simulink model "MPPT_Android"  (R2020a)
settings: Solver=FixedStepAuto  StartTime=0.0  StopTime=0.5  RelTol=1e-3
undefined symbols (not defined in the file): Ion, Lithium
libraries: powerlib x40, androiduilib x6, simulink x2, re_lib x2, powerlib_meascontrol x2, electricdrivelib x1, androidadvancedlib x1
settings Model: Creator=kushalgoswami  LastModifiedBy=kushalgoswami
settings OptimizationCC: EnhancedBackFolding=on  PassReuseOutputArgsAs=Individual arguments  ZeroExternalMemoryAtStartup=off  ZeroInternalMemoryAtStartup=off  MaxStackSize=64  OptimizeBlockOrder=speed  DifferentSizesBufferReuse=on  OptimizationCustomize=off  EfficientTunableParamExpr=on
settings DebuggingCC: ParameterTunabilityLossMsg=error
settings HardwareCC: ProdBitPerPointer=32  ProdBitPerSizeT=32  ProdBitPerPtrDiffT=32  ProdLargestAtomicInteger=Long  ProdLargestAtomicFloat=Double  ProdWordSize=32  ProdHWDeviceType=ARM Compatible->ARM Cortex  UseEmbeddedCoderFeatures=off  UseSimulinkCoderFeatures=off
settings SFSimCC: MATLABDynamicMemAlloc=off
settings RTWCC: SystemTargetFile=ert.tlc  HardwareBoard=Android Device  TemplateMakefile=ert_default_tmf  RTWVerbose=off  Toolchain=Android SDK/NDK Tools
settings CodeAppCC: ForceParamTrailComments=on  IgnoreCustomStorageClasses=off  OperatorAnnotations=on  SimulinkDataObjDesc=on  SFDataObjDesc=on  InsertBlockDesc=on
settings ERTTargetCC: SupportNonInlinedSFcns=on

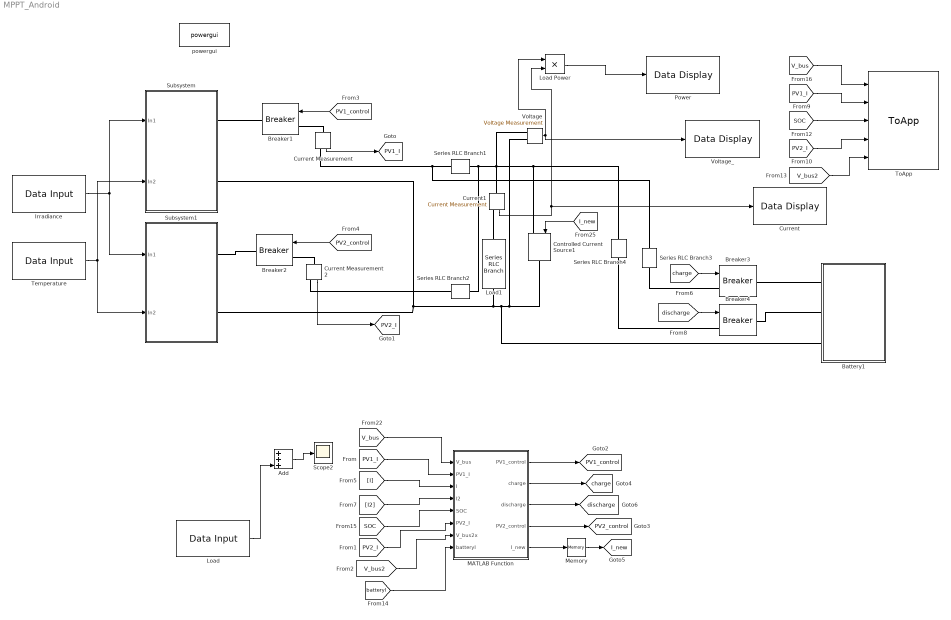
== system MPPT_Android ==
  Add : Sum  Inputs=+++
  Battery1 : Subsystem
  Breaker{1..4} (4 alike) : powerlib/Elements/Breaker  InitialState=0  SwitchingTimes="[1/60  5/60]"  External=on  BreakerResistance=0.01  SnubberResistance=1e6  SnubberCapacitance=inf  Measurements=None  MoreParameters=on  NoBreakLoop=off
  Controlled Current Source1 : powerlib/Electrical Sources/Controlled Current Source  Initialize=off  Source_Type=AC  Amplitude=0  Phase=0  Frequency=0  Measurements=None
  Current : androiduilib/Data Display  DataDisplayId=MPPT_Android/Current  Format=Float  Precision=6  SimulateUsing=Code generation  blockPlatform=Android
      settings: SourceProductBaseCode=ANDROID
  Current Measurement : powerlib/Measurements/Current Measurement  PhasorSimulation=off  OutputType=Complex  PSBequivalent=0
  Current Measurement2 : powerlib/Measurements/Current Measurement  PhasorSimulation=off  OutputType=Complex  PSBequivalent=0
  Current1 : powerlib/Measurements/Current Measurement  PhasorSimulation=off  OutputType=Complex  PSBequivalent=0
  Irradiance : androiduilib/Data Input  isCharVector=off  Value=1000  CharVector=Hello World  OutputDataType=double  maxCharVectorSize=100  DataInputId=MPPT_Android/Irradiance  SampleTime=0.1
      settings: SourceProductBaseCode=ANDROID
  Load : androiduilib/Data Input  isCharVector=off  Value=350  CharVector=Hello World  OutputDataType=double  maxCharVectorSize=100  DataInputId=MPPT_Android/Load  SampleTime=0.1
      settings: SourceProductBaseCode=ANDROID
  Load Power : Product
  Load1 : powerlib/Elements/Series RLC Branch  LConnTagsString=__new0  RConnTagsString=__new0  BranchType=R  Resistance=2  Inductance=1e-3  SetiL0=off  InitialCurrent=0  Capacitance=3300e-6  Setx0=off  InitialVoltage=0  Measurements=None
  MATLAB Function : MATLAB Function  TreatAsAtomicUnit=on
  Memory : Memory
  Power : androiduilib/Data Display  DataDisplayId=MPPT_Android/Power  Format=Float  Precision=6  SimulateUsing=Code generation  blockPlatform=Android
      settings: SourceProductBaseCode=ANDROID
  Scope2 : Scope
  Series RLC Branch{1..4} (4 alike) : powerlib/Elements/Series RLC Branch  LConnTagsString=__new0  RConnTagsString=__new0  BranchType=R  Resistance=0.5  Inductance=1e-3  SetiL0=off  InitialCurrent=0  Capacitance=3300e-6  Setx0=off  InitialVoltage=0  Measurements=None
  Subsystem : Subsystem
      settings: PortSchema="{\"entries\":[{\"content\":{\"sides\":[{\"content\":{\"connectorIds\":[\"LConn1\",\"LConn2\"]},\"type\":\"ConnectorPlacement.EquallySpacedRectSide\",\"uuid\":\"fe52fdc6-6768-4979-b6cd-1f1e64aed3c2\"},{\"content\":{\"connectorIds\":[\"In1\",\"In2\"],\"side\":\"RIGHT\"},\"type\":\"ConnectorPlacement.EquallySpacedRectSide\",\"uuid\":\"5c57de2a-0e2a-4d93-8a44-5c93cac66104\"},{\"content\":{\"connectorIds\":[],\"side\":\"TOP\"},\"type\":\"ConnectorPlacement.EquallySpacedRectSide\",\"uuid\":\"1ec0e451-aef4-49c0-8277-43179a2299e6\"}]},\"type\":\"ConnectorPlacement.EquallySpacedConnector\",\"uuid\":\"46266059-5c92-4136-9283-09609ad0783e\"}],\"packageUris\":[\"http://schema.mathworks.com/mf0/Connector/19700101\"],\"version\":\"1.0\"}"
  Subsystem1 : Subsystem
      settings: PortSchema="{\"entries\":[{\"content\":{\"sides\":[{\"content\":{\"connectorIds\":[\"LConn1\",\"LConn2\"]},\"type\":\"ConnectorPlacement.EquallySpacedRectSide\",\"uuid\":\"fe52fdc6-6768-4979-b6cd-1f1e64aed3c2\"},{\"content\":{\"connectorIds\":[\"In1\",\"In2\"],\"side\":\"RIGHT\"},\"type\":\"ConnectorPlacement.EquallySpacedRectSide\",\"uuid\":\"5c57de2a-0e2a-4d93-8a44-5c93cac66104\"},{\"content\":{\"connectorIds\":[],\"side\":\"TOP\"},\"type\":\"ConnectorPlacement.EquallySpacedRectSide\",\"uuid\":\"1ec0e451-aef4-49c0-8277-43179a2299e6\"}]},\"type\":\"ConnectorPlacement.EquallySpacedConnector\",\"uuid\":\"46266059-5c92-4136-9283-09609ad0783e\"}],\"packageUris\":[\"http://schema.mathworks.com/mf0/Connector/19700101\"],\"version\":\"1.0\"}"
  Temperature : androiduilib/Data Input  isCharVector=off  Value=25  CharVector=Hello World  OutputDataType=double  maxCharVectorSize=100  DataInputId=MPPT_Android/Temperature  SampleTime=0.1
      settings: SourceProductBaseCode=ANDROID
  ToApp : androidadvancedlib/ToApp  FunctionName=ToAppMethod  NumInputs=5
      settings: SourceProductBaseCode=ANDROID
  Voltage : powerlib/Measurements/Voltage Measurement  PhasorSimulation=off  OutputType=Complex  PSBequivalent=0
  Voltage_ : androiduilib/Data Display  DataDisplayId=MPPT_Android/Voltage_  Format=Float  Precision=6  SimulateUsing=Code generation  blockPlatform=Android
      settings: SourceProductBaseCode=ANDROID
  powergui : powerlib/powergui  Priority=1  SimulationMode=Discrete  SampleTime=1e-6  frequency=60  Iterations=50  frequencyindice=0  Pbase=100e6  ErrMax=1e-4  UnitsV=kV  UnitsW=MW  buscounter=0  FunctionMessages=off  echomessages=off  EnableUseOfTLC=off  CurrentSourceSwitches=off  DisableSnubberDevices=off  DisableRonSwitches=off  DisableVfSwitches=off  DisplayEquations=off  AutomaticDiscreteSolvers=off  SolverType=Tustin/Backward Euler (TBE)  Interpol=off  ExternalGateDelay=off  methode=off  Ts=100  x0status=blocks  SPID=on  SwTol=0  HookPort=off  NonlinearTolerance=1e-4  nMaxIteration=100  ContinueOnMaxIteration=off  RestoreLinks=warning  ResistiveCurrentMeasurement=off  Frange=[0:2:500]  Ylog=off  Xlog=on  ShowGrid=off  save=off  variable=ZData  structure=0  ZoomFFT=off  StartTime=0.0  cycles=1  DisplayStyle=1  fundamental=60  FreqAxis=off  MaxFrequency=1000  frequencyindicesteady=1  RmsSteady=1  display=off
  tag scope: I_new=global, PV1_I=global, PV1_control=global, PV2_I=global, PV2_control=global, charge=global, discharge=global
  wires:
  MATLAB Function/3(discharge) -> [discharge]
  [batteryI] -> MATLAB Function/8(batteryI)
  MATLAB Function/5(I_new) -> Memory/1
  [PV2_I] -> MATLAB Function/6(PV2_I)
  [I] -> MATLAB Function/3(I)
  [PV1_I] -> MATLAB Function/2(PV1_I)
  [V_bus2] -> MATLAB Function/7(V_bus2x)
  MATLAB Function/2(charge) -> [charge]
  [I2] -> MATLAB Function/4(I2)
  [SOC] -> MATLAB Function/5(SOC)
  Memory/1 -> [I_new]
  Voltage/1 -> Load Power/1, Voltage_/1
  Current1/1 -> Load Power/2, Current/1
  Current Measurement/1 -> [PV1_I]
  [discharge] -> Breaker4/1
  MATLAB Function/4(PV2_control) -> [PV2_control]
  Load Power/1 -> Power/1
  Current Measurement2/1 -> [PV2_I]
  [V_bus] -> MATLAB Function/1(V_bus)
  [charge] -> Breaker3/1
  [PV1_control] -> Breaker1/1
  [PV2_control] -> Breaker2/1
  [I_new] -> Controlled Current Source1/1
  MATLAB Function/1(PV1_control) -> [PV1_control]
  ? -> Add/1
  ? -> Add/2
  Load/1 -> Add/3
  Add/1 -> Scope2/1
  Irradiance/1 -> Subsystem1/1(In1), Subsystem/1(In1)
  Temperature/1 -> Subsystem1/2(In2), Subsystem/2(In2)
  [SOC] -> ToApp/3
  [PV1_I] -> ToApp/2
  [V_bus] -> ToApp/1
  [PV2_I] -> ToApp/4
  [V_bus2] -> ToApp/5
  connections:
  Series RLC Branch1/LConn1 -- Current1/LConn1 -- Voltage/LConn1 -- Series RLC Branch4/RConn1 -- Controlled Current Source1/LConn1 -- Series RLC Branch2/LConn1
  Battery1/LConn3 -- Subsystem/LConn2 -- Subsystem1/LConn2 -- Load1/RConn1 -- Controlled Current Source1/RConn1 -- Voltage/LConn2
  Series RLC Branch3/RConn1 -- Current Measurement/RConn1 -- Series RLC Branch1/RConn1
  Breaker4/RConn1 -- Battery1/LConn2
  Breaker1/LConn1 -- Current Measurement/LConn1
  Breaker4/LConn1 -- Series RLC Branch4/LConn1
  Subsystem/LConn1 -- Breaker1/RConn1
  Series RLC Branch2/RConn1 -- Current Measurement2/RConn1
  Subsystem1/LConn1 -- Breaker2/RConn1
  Breaker2/LConn1 -- Current Measurement2/LConn1
  Breaker3/LConn1 -- Series RLC Branch3/LConn1
  Breaker3/RConn1 -- Battery1/LConn1
  Current1/RConn1 -- Load1/LConn1

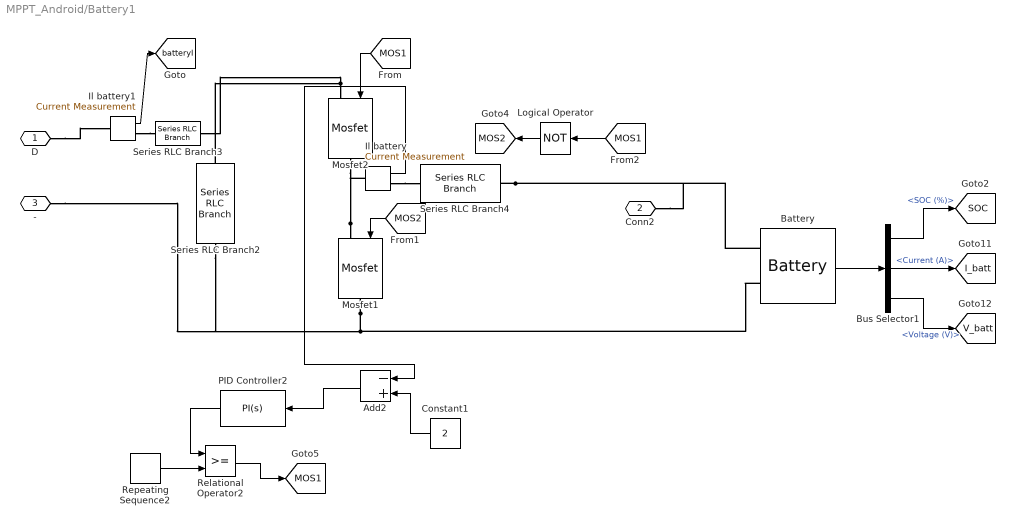
== system MPPT_Android/Battery1 ==
  Add2 : Sum  Inputs=-+
  Battery : electricdrivelib/Extra Sources/Battery  BatType=Lithium-Ion  ShowTempParam=off  ThermalPreset=no  ShowAgeParam=off  NomV=24  NomQ=10  SOC=80  Batt_Tr=0.01  PresetModel=on  MaxQ=10  MinV=18  FullV=27.9357  Dis_rate=4.3478  R=0.024  Normal_OP=9.0435  expZone="[25.9293     0.491304]"  current=[6.5 13 32.5]  Units=Time  Tci=20  NomT=20  T2=-30  MaxQ2=4.8  FullV2=7.1  Normal_OP2=5.655  expZone2="[6.58           1]"  Rca=0.6  ti=2000  Dp=0  Neq0=0  Tsim=1e6  Ta1=25  Qeol=5.4*0.9  Reol=0.013333*1.2  Char_age=[2.3478, 3]  Dis_age=[2.3478, 10]  N1=1500  N2=10500  N3=1000  N4=1400  Ta2=45  N5=950
  Bus Selector1 : BusSelector  OutputSignals=SOC (%),Current (A),Voltage (V)
  Constant1 : Constant  Value=2
  Il battery : powerlib/Measurements/Current Measurement  PhasorSimulation=off  OutputType=Complex  PSBequivalent=0
  Il battery1 : powerlib/Measurements/Current Measurement  PhasorSimulation=off  OutputType=Complex  PSBequivalent=0
  Logical Operator : Logic  Operator=NOT  IconShape=distinctive  AllPortsSameDT=off  OutDataTypeStr=boolean
  Mosfet1 : powerlib/Power Electronics/Mosfet  Ron=0.1  Lon=0  Rd=0.01  Vfd=0  IC=0  Rs=1e5  Cs=inf  Measurements=off
  Mosfet2 : powerlib/Power Electronics/Mosfet  Ron=0.1  Lon=0  Rd=0.01  Vfd=0  IC=0  Rs=1e5  Cs=inf  Measurements=off
  PID Controller2 : simulink/Continuous/PID Controller  Controller=PI  Form=Ideal  TimeDomain=Continuous-time  UseExternalTs=off  SampleTime=-1  IntegratorMethod=Forward Euler  FilterMethod=Forward Euler  ControllerParametersSource=internal  P=0.7  I=100  D=0  UseFilter=on  N=100  TunerSelectOption=Transfer Function Based (PID Tuner App)  InitialConditionSource=internal  InitialConditionForIntegrator=0  InitialConditionForFilter=0  DifferentiatorICPrevScaledInput=0  ExternalReset=none  TrackingMode=off  Kt=1  LimitOutput=on  UpperSaturationLimit=0.9  LowerSaturationLimit=0  LinearizeAsGain=on  AntiWindupMode=none  Kb=1  POutMin=[]  POutMax=[]  IOutMin=[]  IOutMax=[]  DOutMin=[]  DOutMax=[]  NOutMin=[]  NOutMax=[]  SumOutMin=[]  SumOutMax=[]  SaturationOutMin=[]  SaturationOutMax=[]  PParamMin=[]  PParamMax=[]  IParamMin=[]  IParamMax=[]  DParamMin=[]  DParamMax=[]  NParamMin=[]  NParamMax=[]  KbParamMin=[]  KbParamMax=[]  KtParamMin=[]  KtParamMax=[]  KbOutMin=[]  KbOutMax=[]  KtOutMin=[]  KtOutMax=[]  IntegratorOutMin=[]  IntegratorOutMax=[]  FilterOutMin=[]  FilterOutMax=[]  SumI1OutMin=[]  SumI1OutMax=[]  SumI2OutMin=[]  SumI2OutMax=[]  SumI3OutMin=[]  SumI3OutMax=[]  SumI4OutMin=[]  SumI4OutMax=[]  SumDOutMin=[]  SumDOutMax=[]  DifferentiatorOutMin=[]  DifferentiatorOutMax=[]  FilterDiffOutCoefMin=[]  FilterDiffOutCoefMax=[]  ReciprocalOutMin=[]  ReciprocalOutMax=[]  SumDenOutMin=[]  SumDenOutMax=[]  SumNumOutMin=[]  SumNumOutMax=[]  DivideOutMin=[]  DivideOutMax=[]  UdiffTsProdOutMin=[]  UdiffTsProdOutMax=[]  NTsProdOutMin=[]  NTsProdOutMax=[]  UintegralTsProdOutMin=[]  UintegralTsProdOutMax=[]  UngainTsProdOutMin=[]  UngainTsProdOutMax=[]  IntegratorContinuousStateAttributes=''  IntegratorStateMustResolveToSignalObject=off  IntegratorRTWStateStorageClass=Auto  FilterContinuousStateAttributes=''  FilterStateMustResolveToSignalObject=off  FilterRTWStateStorageClass=Auto  ParallelPVariant=Passthrough  IdealPVariant=InternalParameters  IVariant=InternalParameters  DVariant=Disabled  IntegratorVariant=Continuous  SatVariant=Enabled  AWVariant=Passthrough  PCopyVariant=Disabled  TRVariant=Disabled  FdbkBlocksVariant=Forward  IdealPFdbkVariant=Disabled  SatFdbkVariant=Disabled  DerivativeFilterVariant=Disabled  NVariant=Disabled  NCopyVariant=Disabled_SignalSpec  FilterICVariant=Disabled  IntegratorICVariant=InternalICs  ExternalResetVariant=Disabled  TRSumVariant=Passthrough  SumFdbkVariant=Disabled  SumVariant=Sum_PI  TsampFilterVariant=InternalTs  TsampNgainVariant=Passthrough  TsampIntegralVariant=Passthrough
  Relational Operator2 : RelationalOperator  OutDataTypeStr=boolean  RndMeth=Simplest
  Repeating Sequence2 : simulink/Sources/Repeating Sequence  rep_seq_t=[0 100e-6]  rep_seq_y=[0 1]
  Series RLC Branch2 : powerlib/Elements/Series RLC Branch  LConnTagsString=__new0  RConnTagsString=__new0  BranchType=C  Resistance=0.001  Inductance=5.76e-4  SetiL0=off  InitialCurrent=0  Capacitance=500e-6  Setx0=off  InitialVoltage=0  Measurements=None
  Series RLC Branch3 : powerlib/Elements/Series RLC Branch  LConnTagsString=__new0  RConnTagsString=__new0  BranchType=L  Resistance=0.05  Inductance=20e-6  SetiL0=off  InitialCurrent=0  Capacitance=1e-6  Setx0=off  InitialVoltage=0  Measurements=None
  Series RLC Branch4 : powerlib/Elements/Series RLC Branch  LConnTagsString=__new0  RConnTagsString=__new0  BranchType=RL  Resistance=0.05  Inductance=2e-3  SetiL0=off  InitialCurrent=0  Capacitance=1e-6  Setx0=off  InitialVoltage=0  Measurements=None
  D : PMIOPort  Side=Left
  Conn2 : PMIOPort  Port=2  Side=Left
  - : PMIOPort  Port=3  Side=Left
  tag scope: I_batt=global, MOS1=global, MOS2=global, SOC=global, V_batt=global, batteryI=global
  wires:
  [MOS1] -> Mosfet2/1
  Bus Selector1/1 -> [SOC]  "<SOC (%)>"
  [MOS2] -> Mosfet1/1
  Bus Selector1/3 -> [V_batt]  "<Voltage (V)>"
  Battery/1 -> Bus Selector1/1
  Logical Operator/1 -> [MOS2]
  Bus Selector1/2 -> [I_batt]  "<Current (A)>"
  Il battery/1 -> Add2/1
  Add2/1 -> PID Controller2/1
  Repeating Sequence2/1 -> Relational Operator2/2
  Relational Operator2/1 -> [MOS1]
  [MOS1] -> Logical Operator/1
  Constant1/1 -> Add2/2
  PID Controller2/1 -> Relational Operator2/1
  Il battery1/1 -> [batteryI]
  connections:
  Series RLC Branch4/RConn1 -- Conn2/RConn1 -- Battery/LConn1
  Mosfet1/LConn1 -- Mosfet2/RConn1 -- Il battery/LConn1
  Mosfet1/RConn1 -- Battery/LConn2 -- Series RLC Branch2/RConn1 -- -/RConn1
  Il battery/RConn1 -- Series RLC Branch4/LConn1
  D/RConn1 -- Il battery1/LConn1
  Mosfet2/LConn1 -- Series RLC Branch3/RConn1 -- Series RLC Branch2/LConn1
  Il battery1/RConn1 -- Series RLC Branch3/LConn1

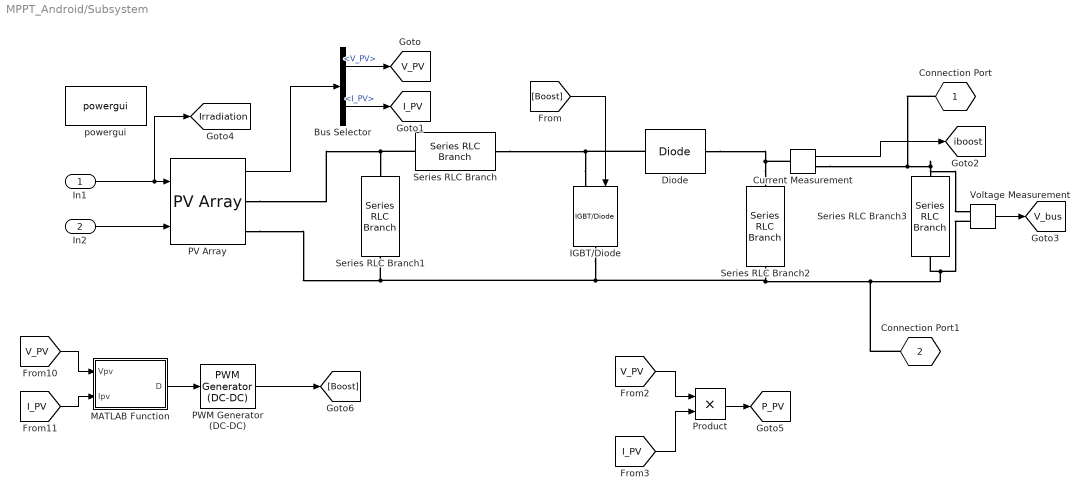
== system MPPT_Android/Subsystem ==
  In1 : Inport
  In2 : Inport  Port=2
  Bus Selector : BusSelector  OutputSignals=V_PV,I_PV
  Current Measurement : powerlib/Measurements/Current Measurement  PhasorSimulation=off  OutputType=Complex  PSBequivalent=0
  Diode : powerlib/Power Electronics/Diode  Ron=0.001  Lon=0  Vf=0.8  IC=0  UseSnubber=0  Rs=500  Cs=250e-9  Measurements=off
  IGBT/Diode : powerlib/Power Electronics/IGBT//Diode  Ron=1e-3  Rs=1e5  Cs=inf  Measurements=off
  MATLAB Function : MATLAB Function  TreatAsAtomicUnit=on
  PV Array : re_lib/Solar/PV Array  Npar=1  Nser=1  PlotType=array @ 1000 W/m2 & specified temperatures  S_vec="[ 1000  500  100 ]"  Temp_C_vec="[ 45 25  ]"  ModuleName=1Soltech 1STH-250-WH  PlotWhenSelected=off  Pm=250.205  Ncell=60  Voc=37.3  Isc=8.66  Vm=30.7  Im=8.15  beta_Voc_pc=-0.36901  alpha_Isc_pc=0.086998  beta_Voc=-0.13764  alpha_Isc=0.007534  IL=8.7106  I0=4.1601e-10  nI=1.019  Rsh=224.1886  Rs=0.23724  RobustModel=off  RobustCellTemperature=25  BAL=on  Tc=1e-6  Tfilter=5e-5
  PWM Generator (DC-DC) : powerlib_meascontrol/Pulse & Signal Generators/PWM Generator (DC-DC)  Fsw=5000  Ts=10e-6
  Product : Product
  Series RLC Branch : powerlib/Elements/Series RLC Branch  LConnTagsString=__new0  RConnTagsString=__new0  BranchType=L  Resistance=0.1  Inductance=5e-3  SetiL0=off  InitialCurrent=0  Capacitance=1e-6  Setx0=off  InitialVoltage=0  Measurements=None
  Series RLC Branch1 : powerlib/Elements/Series RLC Branch  LConnTagsString=__new0  RConnTagsString=__new0  BranchType=C  Resistance=1e-4  Inductance=1e-3  SetiL0=off  InitialCurrent=0  Capacitance=100e-6  Setx0=off  InitialVoltage=0  Measurements=None
  Series RLC Branch2 : powerlib/Elements/Series RLC Branch  LConnTagsString=__new0  RConnTagsString=__new0  BranchType=C  Resistance=1e-4  Inductance=1e-3  SetiL0=off  InitialCurrent=0  Capacitance=3300e-6  Setx0=off  InitialVoltage=0  Measurements=None
  Series RLC Branch3 : powerlib/Elements/Series RLC Branch  LConnTagsString=__new0  RConnTagsString=__new0  BranchType=R  Resistance=10  Inductance=1e-3  SetiL0=off  InitialCurrent=0  Capacitance=3300e-6  Setx0=off  InitialVoltage=0  Measurements=None
  Voltage Measurement : powerlib/Measurements/Voltage Measurement  PhasorSimulation=off  OutputType=Complex  PSBequivalent=0
  powergui : powerlib/powergui  Priority=1  SimulationMode=Discrete  SampleTime=1e-6  frequency=60  Iterations=50  frequencyindice=0  Pbase=100e6  ErrMax=1e-4  UnitsV=kV  UnitsW=MW  buscounter=0  FunctionMessages=off  echomessages=off  EnableUseOfTLC=off  CurrentSourceSwitches=off  DisableSnubberDevices=off  DisableRonSwitches=off  DisableVfSwitches=off  DisplayEquations=off  AutomaticDiscreteSolvers=off  SolverType=Tustin/Backward Euler (TBE)  Interpol=off  ExternalGateDelay=off  methode=off  Ts=100  x0status=blocks  SPID=on  SwTol=0  HookPort=off  NonlinearTolerance=1e-4  nMaxIteration=100  ContinueOnMaxIteration=off  RestoreLinks=warning  ResistiveCurrentMeasurement=off  Frange=[0:2:500]  Ylog=off  Xlog=on  ShowGrid=off  save=off  variable=ZData  structure=0  ZoomFFT=off  StartTime=0.0  cycles=1  DisplayStyle=1  fundamental=60  FreqAxis=off  MaxFrequency=1000  frequencyindicesteady=1  RmsSteady=1  display=off
  Connection Port : PMIOPort  Tag=PMCPort  Side=Left
  Connection Port1 : PMIOPort  Tag=PMCPort  Port=2  Side=Left
  tag scope: I_PV=global, Irradiation=global, P_PV=global, V_PV=global, V_bus=global, iboost=global
  wires:
  Bus Selector/1 -> [V_PV]  "<V_PV>"
  [I_PV] -> MATLAB Function/2(Ipv)
  [I_PV] -> Product/2
  Voltage Measurement/1 -> [V_bus]
  [V_PV] -> Product/1
  Bus Selector/2 -> [I_PV]  "<I_PV>"
  [Boost] -> IGBT/Diode/1
  Current Measurement/1 -> [iboost]
  [V_PV] -> MATLAB Function/1(Vpv)
  In2/1 -> PV Array/2
  PWM Generator (DC-DC)/1 -> [Boost]
  In1/1 -> [Irradiation], PV Array/1
  PV Array/1 -> Bus Selector/1
  MATLAB Function/1(D) -> PWM Generator (DC-DC)/1
  Product/1 -> [P_PV]
  connections:
  Voltage Measurement/LConn2 -- Connection Port1/RConn1 -- IGBT/Diode/RConn1 -- PV Array/RConn2 -- Series RLC Branch1/RConn1 -- Series RLC Branch2/RConn1 -- Series RLC Branch3/RConn1
  Series RLC Branch/LConn1 -- PV Array/RConn1 -- Series RLC Branch1/LConn1
  Series RLC Branch2/LConn1 -- Diode/RConn1 -- Current Measurement/LConn1
  IGBT/Diode/LConn1 -- Series RLC Branch/RConn1 -- Diode/LConn1
  Series RLC Branch3/LConn1 -- Connection Port/RConn1 -- Current Measurement/RConn1 -- Voltage Measurement/LConn1

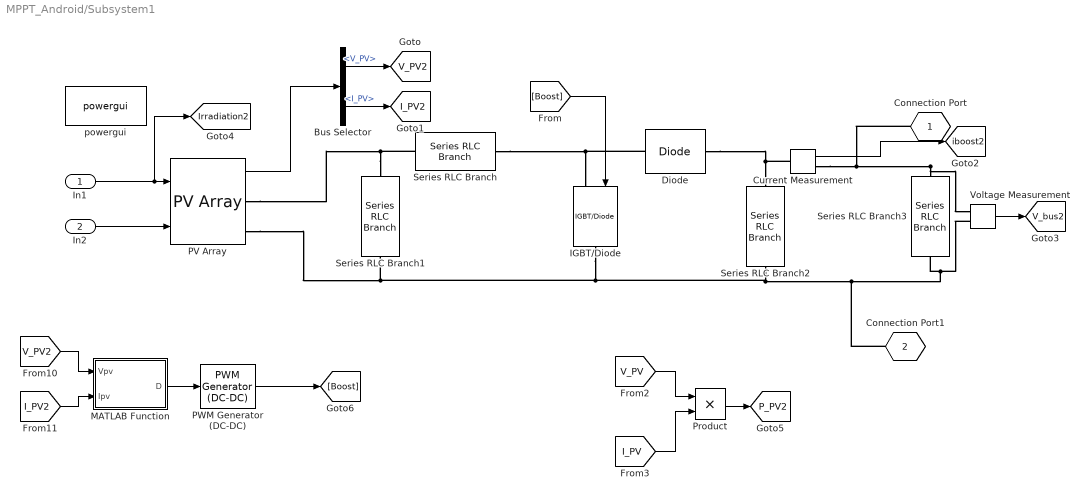
== system MPPT_Android/Subsystem1 ==
  In1 : Inport
  In2 : Inport  Port=2
  Bus Selector : BusSelector  OutputSignals=V_PV,I_PV
  Current Measurement : powerlib/Measurements/Current Measurement  PhasorSimulation=off  OutputType=Complex  PSBequivalent=0
  Diode : powerlib/Power Electronics/Diode  Ron=0.001  Lon=0  Vf=0.8  IC=0  UseSnubber=0  Rs=500  Cs=250e-9  Measurements=off
  IGBT/Diode : powerlib/Power Electronics/IGBT//Diode  Ron=1e-3  Rs=1e5  Cs=inf  Measurements=off
  MATLAB Function : MATLAB Function  TreatAsAtomicUnit=on
  PV Array : re_lib/Solar/PV Array  Npar=1  Nser=1  PlotType=array @ 1000 W/m2 & specified temperatures  S_vec="[ 1000  500  100 ]"  Temp_C_vec="[ 45 25  ]"  ModuleName=1Soltech 1STH-250-WH  PlotWhenSelected=off  Pm=250.205  Ncell=60  Voc=37.3  Isc=8.66  Vm=30.7  Im=8.15  beta_Voc_pc=-0.36901  alpha_Isc_pc=0.086998  beta_Voc=-0.13764  alpha_Isc=0.007534  IL=8.7106  I0=4.1601e-10  nI=1.019  Rsh=224.1886  Rs=0.23724  RobustModel=off  RobustCellTemperature=25  BAL=on  Tc=1e-6  Tfilter=5e-5
  PWM Generator (DC-DC) : powerlib_meascontrol/Pulse & Signal Generators/PWM Generator (DC-DC)  Fsw=5000  Ts=10e-6
  Product : Product
  Series RLC Branch : powerlib/Elements/Series RLC Branch  LConnTagsString=__new0  RConnTagsString=__new0  BranchType=L  Resistance=0.1  Inductance=5e-3  SetiL0=off  InitialCurrent=0  Capacitance=1e-6  Setx0=off  InitialVoltage=0  Measurements=None
  Series RLC Branch1 : powerlib/Elements/Series RLC Branch  LConnTagsString=__new0  RConnTagsString=__new0  BranchType=C  Resistance=1e-4  Inductance=1e-3  SetiL0=off  InitialCurrent=0  Capacitance=100e-6  Setx0=off  InitialVoltage=0  Measurements=None
  Series RLC Branch2 : powerlib/Elements/Series RLC Branch  LConnTagsString=__new0  RConnTagsString=__new0  BranchType=C  Resistance=1e-4  Inductance=1e-3  SetiL0=off  InitialCurrent=0  Capacitance=3300e-6  Setx0=off  InitialVoltage=0  Measurements=None
  Series RLC Branch3 : powerlib/Elements/Series RLC Branch  LConnTagsString=__new0  RConnTagsString=__new0  BranchType=R  Resistance=10  Inductance=1e-3  SetiL0=off  InitialCurrent=0  Capacitance=3300e-6  Setx0=off  InitialVoltage=0  Measurements=None
  Voltage Measurement : powerlib/Measurements/Voltage Measurement  PhasorSimulation=off  OutputType=Complex  PSBequivalent=0
  powergui : powerlib/powergui  Priority=1  SimulationMode=Discrete  SampleTime=1e-6  frequency=60  Iterations=50  frequencyindice=0  Pbase=100e6  ErrMax=1e-4  UnitsV=kV  UnitsW=MW  buscounter=0  FunctionMessages=off  echomessages=off  EnableUseOfTLC=off  CurrentSourceSwitches=off  DisableSnubberDevices=off  DisableRonSwitches=off  DisableVfSwitches=off  DisplayEquations=off  AutomaticDiscreteSolvers=off  SolverType=Tustin/Backward Euler (TBE)  Interpol=off  ExternalGateDelay=off  methode=off  Ts=100  x0status=blocks  SPID=on  SwTol=0  HookPort=off  NonlinearTolerance=1e-4  nMaxIteration=100  ContinueOnMaxIteration=off  RestoreLinks=warning  ResistiveCurrentMeasurement=off  Frange=[0:2:500]  Ylog=off  Xlog=on  ShowGrid=off  save=off  variable=ZData  structure=0  ZoomFFT=off  StartTime=0.0  cycles=1  DisplayStyle=1  fundamental=60  FreqAxis=off  MaxFrequency=1000  frequencyindicesteady=1  RmsSteady=1  display=off
  Connection Port : PMIOPort  Tag=PMCPort  Side=Left
  Connection Port1 : PMIOPort  Tag=PMCPort  Port=2  Side=Left
  tag scope: I_PV2=global, Irradiation2=global, P_PV2=global, V_PV2=global, V_bus2=global, iboost2=global
  wires:
  Bus Selector/1 -> [V_PV2]  "<V_PV>"
  [I_PV2] -> MATLAB Function/2(Ipv)
  [I_PV] -> Product/2
  Voltage Measurement/1 -> [V_bus2]
  [V_PV] -> Product/1
  Bus Selector/2 -> [I_PV2]  "<I_PV>"
  [Boost] -> IGBT/Diode/1
  Current Measurement/1 -> [iboost2]
  [V_PV2] -> MATLAB Function/1(Vpv)
  In2/1 -> PV Array/2
  PWM Generator (DC-DC)/1 -> [Boost]
  In1/1 -> [Irradiation2], PV Array/1
  PV Array/1 -> Bus Selector/1
  MATLAB Function/1(D) -> PWM Generator (DC-DC)/1
  Product/1 -> [P_PV2]
  connections:
  Voltage Measurement/LConn2 -- Connection Port1/RConn1 -- PV Array/RConn2 -- Series RLC Branch1/RConn1 -- IGBT/Diode/RConn1 -- Series RLC Branch2/RConn1 -- Series RLC Branch3/RConn1
  Series RLC Branch1/LConn1 -- Series RLC Branch/LConn1 -- PV Array/RConn1
  Current Measurement/LConn1 -- Series RLC Branch2/LConn1 -- Diode/RConn1
  Diode/LConn1 -- IGBT/Diode/LConn1 -- Series RLC Branch/RConn1
  Current Measurement/RConn1 -- Series RLC Branch3/LConn1 -- Voltage Measurement/LConn1 -- Connection Port/RConn1

== matlab function MPPT_Android/Subsystem1/MATLAB Function ==
  data: Vpv input; D output; Ipv input
function D = PO(Vpv,Ipv)

Dinit=0.42;
Dmax=0.8;
Dmin=0.08;
deltaD=0.000005;

persistent Dprev Pprev Vprev

if isempty(Vprev)
    Vprev=0;
    Dprev=Dinit;
    Pprev=0;
end

deltaD=125e-6;

Ppv=Vpv*Ipv;

if (Ppv-Pprev)~=0
    if (Ppv-Pprev)>0
        if (Vpv-Vprev)>0
            D=Dprev-deltaD;
        else
            D=Dprev+deltaD;
        end
    else
        if (Vpv-Vprev)>0
            D=Dprev+deltaD;
        else
            D=Dprev-deltaD;
        end
    end
else
    D=Dprev;
end

if D>=Dmax | D<=Dmin
    D=Dprev;
end
Dprev=D;
Vprev=Vpv;
Pprev=Ppv;

== matlab function MPPT_Android/Subsystem/MATLAB Function ==
  data: Vpv input; D output; Ipv input
function D = PO(Vpv,Ipv)

Dinit=0.42;
Dmax=0.8;
Dmin=0.08;
deltaD=0.000005;

persistent Dprev Pprev Vprev

if isempty(Vprev)
    Vprev=0;
    Dprev=Dinit;
    Pprev=0;
end

deltaD=125e-6;

Ppv=Vpv*Ipv;

if (Ppv-Pprev)~=0
    if (Ppv-Pprev)>0
        if (Vpv-Vprev)>0
            D=Dprev-deltaD;
        else
            D=Dprev+deltaD;
        end
    else
        if (Vpv-Vprev)>0
            D=Dprev+deltaD;
        else
            D=Dprev-deltaD;
        end
    end
else
    D=Dprev;
end

if D>=Dmax | D<=Dmin
    D=Dprev;
end
Dprev=D;
Vprev=Vpv;
Pprev=Ppv;

== matlab function MPPT_Android/MATLAB Function ==
  data: V_bus input; PV1_I input; I input; I2 input; SOC input; PV1_control output; charge output; discharge output; PV2_I input; V_bus2x input; PV2_control output; I_new output; batteryI input
function [PV1_control, charge, discharge, PV2_control, I_new] = fcn(V_bus, PV1_I, I, I2, SOC, PV2_I, V_bus2x, batteryI)
% I - the MPPT reference command from PV-1
% I =  I-PV1 at steady state
R=100;
I_new = I+I2-V_bus2x/R-batteryI;

% Initial state of switches
PV1_control=1;
PV2_control=0;
charge=0;
discharge=0;
load=350;
% Only PV1 is sufficient & battery charging
if V_bus*PV1_I>load && SOC<90
    charge=1;
end

% PV2 also required & battery charging
if V_bus*PV1_I<load
    PV2_control=1;
    charge=1;
end

% Battery also required
if (V_bus*PV1_I)+(V_bus2x*PV2_I)<load && SOC>15
    discharge=1;
    charge=0;
end
